simulink model "torqueBalancingStandup"  (Simulink 8.8)
settings: Solver=FixedStepDiscrete  StartTime=0.0  StopTime="Config.SIMULATION_TIME "  FixedStep=Config.Ts  RelTol=1e-3  EnableMultiTasking=on
InitFcn:
  | cd(fileparts(which(bdroot)));
  | initTorqueBalancingStandup;
StopFcn:
  | cd(fileparts(which(bdroot)));
  | stopTorqueBalancingStandup;
undefined symbols (not defined in the file or in its folder): bVectorConstraintsFeet, bVectorConstraintsLegs, Config, ConstraintsMatrixFeet, ConstraintsMatrixLegs, Gain, HUMAN_DOF_FOR_SIMULINK, Reg, ROBOT_DOF, ROBOT_DOF_FOR_SIMULINK, Sat, Sm
libraries: WBToolboxLibrary x128, simulink x4
(part 1 of 3)
settings Model: SuppressorTable=22 serialization::archive 11 0 3 0 0 0 11 0  Creator=daniele  LastModifiedBy=yeshi  NumberOfSteps=100
settings DataIOCC: SignalLoggingSaveFormat=Dataset
settings OptimizationCC: ExpressionDepthLimit=2147483647
settings DebuggingCC: SolverPrmCheckMsg=warning  AllowSymbolicDim=off
settings SFSimCC: SimParseCustomCode=off

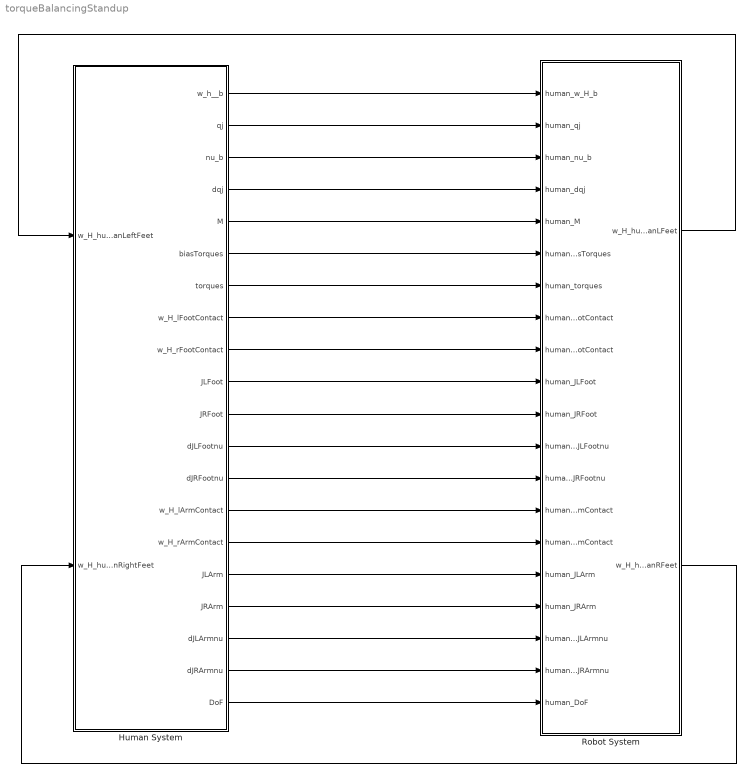
== system torqueBalancingStandup ==
  Human System : Subsystem
  Robot System : Subsystem
  wires:
  Human System/15(w_H_rArmContact) -> Robot System/15(human_w_H_rArmContact)
  Human System/8(w_H_lFootContact) -> Robot System/8(human_w_H_lFootContact)
  Human System/9(w_H_rFootContact) -> Robot System/9(human_w_H_rFootContact)
  Human System/17(JRArm) -> Robot System/17(human_JRArm)
  Human System/19(dJRArmnu) -> Robot System/19(human_dJRArmnu)
  Human System/14(w_H_lArmContact) -> Robot System/14(human_w_H_lArmContact)
  Human System/11(JRFoot) -> Robot System/11(human_JRFoot)
  Human System/12(dJLFootnu) -> Robot System/12(human_dJLFootnu)
  Human System/18(dJLArmnu) -> Robot System/18(human_dJLArmnu)
  Human System/13(dJRFootnu) -> Robot System/13(human_dJRFootnu)
  Human System/1(w_h__b) -> Robot System/1(human_w_H_b)
  Human System/2(qj) -> Robot System/2(human_qj)
  Human System/3(nu_b) -> Robot System/3(human_nu_b)
  Human System/4(dqj) -> Robot System/4(human_dqj)
  Human System/5(M) -> Robot System/5("human_M ")
  Human System/6(biasTorques) -> Robot System/6("human_biasTorques ")
  Human System/10(JLFoot) -> Robot System/10(human_JLFoot)
  Human System/16(JLArm) -> Robot System/16(human_JLArm)
  Human System/7(torques) -> Robot System/7(human_torques)
  Human System/20(DoF) -> Robot System/20(human_DoF)
  Robot System/1(w_H_humanLFeet) -> Human System/1(w_H_humanLeftFeet)
  Robot System/2(w_H_humanRFeet) -> Human System/2(w_H_humanRightFeet)

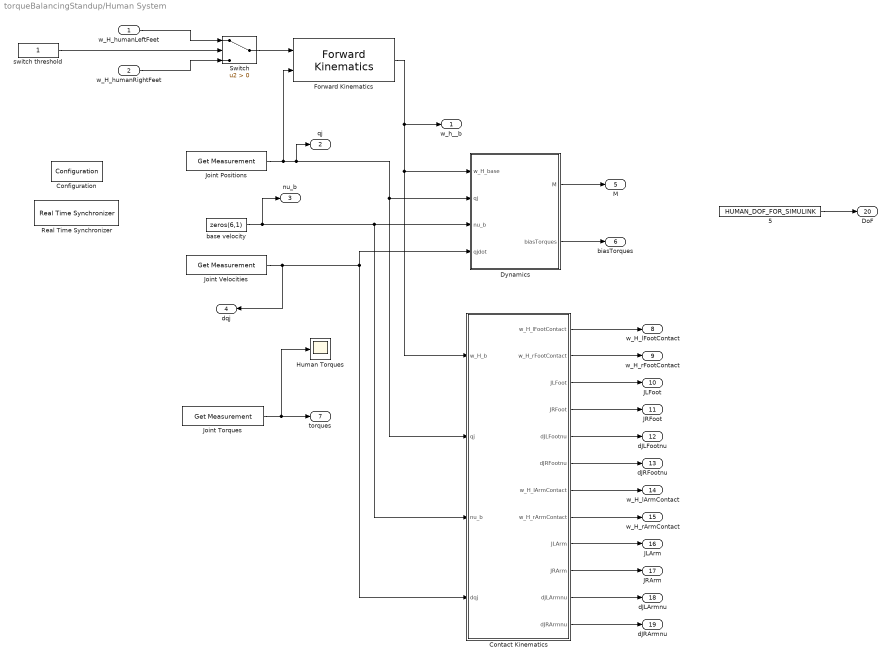
== system torqueBalancingStandup/Human System ==
  w_H_humanLeftFeet : Inport
  w_H_humanRightFeet : Inport  Port=2
  "    5" : Constant  Value=HUMAN_DOF_FOR_SIMULINK
  Configuration : WBToolboxLibrary/Utilities/Configuration  ConfigSource=Workspace  ConfigObject='HUMAN_WBTConfigRobot'
  Contact Kinematics : Subsystem
  Dynamics : Subsystem
  Forward Kinematics : WBToolboxLibrary/wholeBodyModel/Kinematics/Forward Kinematics  frameName=HUMAN_Frames.BASE
  Human Torques : Scope
  Joint Positions : WBToolboxLibrary/wholeBodyStates/Get Measurement  measuredType=Joints Position
  Joint Torques : WBToolboxLibrary/wholeBodyStates/Get Measurement  measuredType=Joints Torque
  Joint Velocities : WBToolboxLibrary/wholeBodyStates/Get Measurement  measuredType=Joints Velocity
  Real Time Synchronizer : WBToolboxLibrary/Utilities/Real Time Synchronizer  period=0.01  mask(Real Time Synchronizer){}
  Switch : Switch  Criteria=u2 > Threshold
  base velocity : Constant  Value=zeros(6,1)
  switch threshold : Constant
  w_h__b : Outport
  qj : Outport  Port=2
  nu_b : Outport  Port=3
  dqj : Outport  Port=4
  M : Outport  Port=5
  biasTorques : Outport  Port=6
  torques : Outport  Port=7
  w_H_lFootContact : Outport  Port=8
  w_H_rFootContact : Outport  Port=9
  JLFoot : Outport  Port=10
  JRFoot : Outport  Port=11
  dJLFootnu : Outport  Port=12
  dJRFootnu : Outport  Port=13
  w_H_lArmContact : Outport  Port=14
  w_H_rArmContact : Outport  Port=15
  JLArm : Outport  Port=16
  JRArm : Outport  Port=17
  dJLArmnu : Outport  Port=18
  dJRArmnu : Outport  Port=19
  DoF : Outport  Port=20
  wires:
  Joint Positions/1 -> Dynamics/2(qj), Contact Kinematics/2(qj), qj/1, Forward Kinematics/2
  base velocity/1 -> nu_b/1, Dynamics/3(nu_b), Contact Kinematics/3(nu_b)
  Joint Velocities/1 -> dqj/1, Dynamics/4(qjdot), Contact Kinematics/4(dqj)
  Forward Kinematics/1 -> w_h__b/1, Contact Kinematics/1(w_H_b), Dynamics/1(w_H_base)
  Dynamics/1(M) -> M/1
  Dynamics/2(biasTorques) -> biasTorques/1
  Contact Kinematics/1(w_H_lFootContact) -> w_H_lFootContact/1
  Contact Kinematics/2(w_H_rFootContact) -> w_H_rFootContact/1
  Contact Kinematics/3(JLFoot) -> JLFoot/1
  Contact Kinematics/4(JRFoot) -> JRFoot/1
  Contact Kinematics/5(dJLFootnu) -> dJLFootnu/1
  Contact Kinematics/6(dJRFootnu) -> dJRFootnu/1
  Contact Kinematics/7(w_H_lArmContact) -> w_H_lArmContact/1
  Contact Kinematics/8(w_H_rArmContact) -> w_H_rArmContact/1
  Contact Kinematics/9(JLArm) -> JLArm/1
  Contact Kinematics/10(JRArm) -> JRArm/1
  Contact Kinematics/11(dJLArmnu) -> dJLArmnu/1
  Contact Kinematics/12(dJRArmnu) -> dJRArmnu/1
  Joint Torques/1 -> Human Torques/1, torques/1
  "    5"/1 -> DoF/1
  w_H_humanRightFeet/1 -> Switch/3
  Switch/1 -> Forward Kinematics/1
  w_H_humanLeftFeet/1 -> Switch/1
  switch threshold/1 -> Switch/2

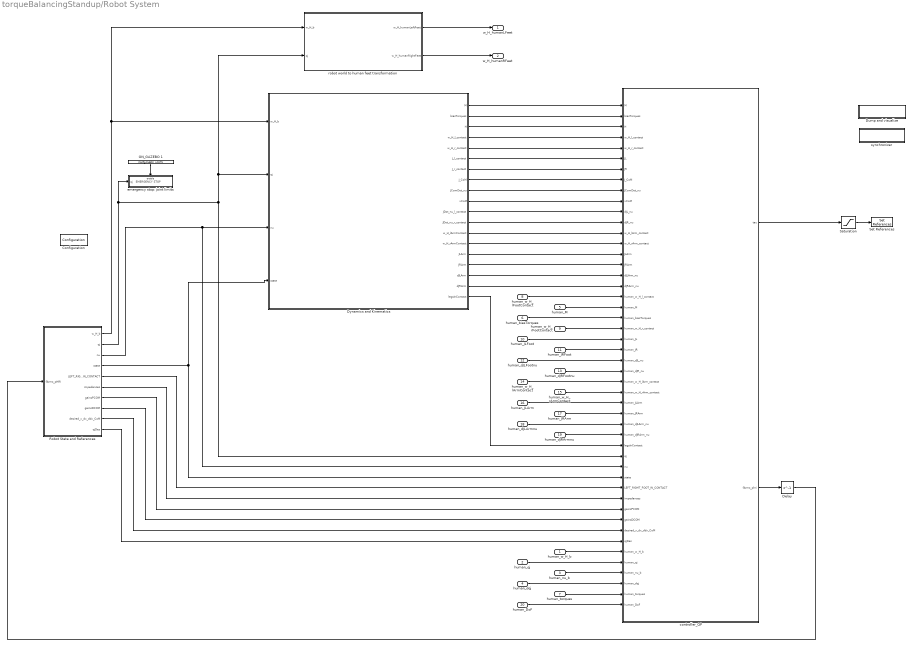
== system torqueBalancingStandup/Robot System ==
  human_w_H_b : Inport
  human_qj : Inport  Port=2
  human_nu_b : Inport  Port=3
  human_dqj : Inport  Port=4
  "human_M " : Inport  Port=5
  "human_biasTorques " : Inport  Port=6
  human_torques : Inport  Port=7
  human_w_H_lFootContact : Inport  Port=8
  human_w_H_rFootContact : Inport  Port=9
  human_JLFoot : Inport  Port=10
  human_JRFoot : Inport  Port=11
  human_dJLFootnu : Inport  Port=12
  human_dJRFootnu : Inport  Port=13
  human_w_H_lArmContact : Inport  Port=14
  human_w_H_rArmContact : Inport  Port=15
  human_JLArm : Inport  Port=16
  human_JRArm : Inport  Port=17
  human_dJLArmnu : Inport  Port=18
  human_dJRArmnu : Inport  Port=19
  human_DoF : Inport  Port=20
  Configuration : WBToolboxLibrary/Utilities/Configuration  ConfigSource=Workspace  ConfigObject='WBTConfigRobot'
  Delay : Delay  DelayLength=1
  Dump and visualize : Subsystem
      mask Display: disp('VISUALIZER')
  Dynamics and Kinematics : Subsystem
  ON_GAZEBO 1 : Constant  Value=Config.CHECK_LIMITS
  Robot State and References : Subsystem  Priority=-10
  Saturation : Saturate  UpperLimit=Sat.torque  LowerLimit=-Sat.torque
  Set References : WBToolboxLibrary/wholeBodyActuators/Set References  controlType=Torque  refSpeed=50
  controller_QP : Subsystem
  emergency stop: joint limits : Subsystem
  robot world to human feet transformation : Subsystem
  synchronizer : Subsystem
      mask Display: disp('SYNCHRONIZER')
  w_H_humanLFeet : Outport
  w_H_humanRFeet : Outport  Port=2
  wires:
  ON_GAZEBO 1/1 -> emergency stop: joint limits/Enable
  Saturation/1 -> Set References/1
  Robot State and References/2(qj) -> controller_QP/34(qj), Dynamics and Kinematics/2(qj), robot world to human feet transformation/2(qj), emergency stop: joint limits/1(qj   EMERGENCY STOP)
  Robot State and References/3(nu) -> Dynamics and Kinematics/3(nu), controller_QP/35(nu)
  Robot State and References/4(state) -> controller_QP/36(state), Dynamics and Kinematics/4("state ")
  Robot State and References/1(w_H_b) -> robot world to human feet transformation/1(w_H_b), Dynamics and Kinematics/1(w_H_b)
  Dynamics and Kinematics/1(M) -> controller_QP/1(M)
  "human_M "/1 -> controller_QP/20(human_M)
  "human_biasTorques "/1 -> controller_QP/21(human_biasTorques)
  Dynamics and Kinematics/2(biasTorques) -> controller_QP/2(biasTorques)
  Dynamics and Kinematics/3(H) -> controller_QP/3("H ")
  Dynamics and Kinematics/4(w_H_l_contact) -> controller_QP/4(w_H_l_contact)
  Dynamics and Kinematics/5(w_H_r_contact) -> controller_QP/5(w_H_r_contact)
  Dynamics and Kinematics/6(J_l_contact) -> controller_QP/6(JL)
  Dynamics and Kinematics/7(J_r_contact) -> controller_QP/7(JR)
  Dynamics and Kinematics/8(J_CoM) -> controller_QP/8(J_CoM)
  Dynamics and Kinematics/10(xCoM) -> controller_QP/10(xCoM)
  Dynamics and Kinematics/11(JDot_nu_l_contact) -> controller_QP/11(dJL_nu)
  Dynamics and Kinematics/12(JDot_nu_r_contact) -> controller_QP/12(dJR_nu)
  Dynamics and Kinematics/13(w_H_lArmContact) -> controller_QP/13(w_H_lArm_contact)
  Dynamics and Kinematics/14(w_H_rArmContact) -> controller_QP/14(w_H_rArm_contact)
  Dynamics and Kinematics/15(JLArm) -> controller_QP/15(JLArm)
  Dynamics and Kinematics/16(JRArm) -> controller_QP/16(JRArm)
  Dynamics and Kinematics/17(dJLArm) -> controller_QP/17(dJLArm_nu)
  Dynamics and Kinematics/18(dJRArm) -> controller_QP/18(dJRArm_nu)
  Dynamics and Kinematics/19(legsInContact) -> controller_QP/33(legsInContact)
  human_w_H_lFootContact/1 -> controller_QP/19(human_w_H_l_contact)
  human_w_H_rFootContact/1 -> controller_QP/22(human_w_H_r_contact)
  human_JLFoot/1 -> controller_QP/23(human_JL)
  human_JRFoot/1 -> controller_QP/24(human_JR)
  human_dJLFootnu/1 -> controller_QP/25(human_dJL_nu)
  human_dJRFootnu/1 -> controller_QP/26(human_dJR_nu)
  human_w_H_lArmContact/1 -> controller_QP/27(human_w_H_lArm_contact)
  human_w_H_rArmContact/1 -> controller_QP/28(human_w_H_rArm_contact)
  human_JLArm/1 -> controller_QP/29(human_JLArm)
  human_JRArm/1 -> controller_QP/30(human_JRArm)
  human_dJLArmnu/1 -> controller_QP/31(human_dJLArm_nu)
  human_dJRArmnu/1 -> controller_QP/32(human_dJRArm_nu)
  controller_QP/1("tau ") -> Saturation/1
  Robot State and References/5(LEFT_RIGHT_FOOT_IN_CONTACT) -> controller_QP/37(LEFT_RIGHT_FOOT_IN_CONTACT)
  Robot State and References/6(impedances) -> controller_QP/38(impedances)
  Robot State and References/7(gainsPCOM) -> controller_QP/39(gainsPCOM)
  Robot State and References/8(gainsDCOM) -> controller_QP/40(gainsDCOM)
  Robot State and References/9(desired_x_dx_ddx_CoM) -> controller_QP/41(desired_x_dx_ddx_CoM)
  Robot State and References/10(qjDes) -> controller_QP/42(qjDes)
  human_w_H_b/1 -> controller_QP/43(human_w_H_b)
  human_qj/1 -> controller_QP/44(human_qj)
  human_nu_b/1 -> controller_QP/45(human_nu_b)
  human_dqj/1 -> controller_QP/46(human_dqj)
  human_torques/1 -> controller_QP/47(human_torques)
  human_DoF/1 -> controller_QP/48(human_DoF)
  robot world to human feet transformation/1(w_H_humanLeftFeet) -> w_H_humanLFeet/1
  robot world to human feet transformation/2(w_H_humanRightFeet) -> w_H_humanRFeet/1
  Dynamics and Kinematics/9(JComDot_nu) -> controller_QP/9(JComDot_nu)
  controller_QP/2(fArms_phri) -> Delay/1
  Delay/1 -> Robot State and References/1(fArms_pHRI)

== system torqueBalancingStandup/Human System/Contact Kinematics ==
  w_H_b : Inport
  qj : Inport  Port=2
  nu_b : Inport  Port=3
  dqj : Inport  Port=4
  Arm Contacts Kinematics : Subsystem
  Leg Contacts Kinematics : Subsystem
  w_H_lFootContact : Outport
  w_H_rFootContact : Outport  Port=2
  JLFoot : Outport  Port=3
  JRFoot : Outport  Port=4
  dJLFootnu : Outport  Port=5
  dJRFootnu : Outport  Port=6
  w_H_lArmContact : Outport  Port=7
  w_H_rArmContact : Outport  Port=8
  JLArm : Outport  Port=9
  JRArm : Outport  Port=10
  dJLArmnu : Outport  Port=11
  dJRArmnu : Outport  Port=12
  wires:
  Arm Contacts Kinematics/3(JLArm) -> JLArm/1
  Arm Contacts Kinematics/5(dJLArmnu) -> dJLArmnu/1
  Leg Contacts Kinematics/3(JLFoot) -> JLFoot/1
  Arm Contacts Kinematics/6(dJRArmnu) -> dJRArmnu/1
  w_H_b/1 -> Arm Contacts Kinematics/1(w_H_b1), Leg Contacts Kinematics/1(w_H_b1)
  nu_b/1 -> Arm Contacts Kinematics/3(nu_b), Leg Contacts Kinematics/3(nu_b)
  Leg Contacts Kinematics/1(w_H_lFootContact) -> w_H_lFootContact/1
  Leg Contacts Kinematics/6(dJRFootnu) -> dJRFootnu/1
  Leg Contacts Kinematics/4(JRFoot) -> JRFoot/1
  Leg Contacts Kinematics/5(dJLFootnu) -> dJLFootnu/1
  Arm Contacts Kinematics/1(w_H_lArmContact) -> w_H_lArmContact/1
  dqj/1 -> Arm Contacts Kinematics/4(dqj), Leg Contacts Kinematics/4(dqj)
  Leg Contacts Kinematics/2(w_H_rFootContact) -> w_H_rFootContact/1
  Arm Contacts Kinematics/2(w_H_rArmContact) -> w_H_rArmContact/1
  Arm Contacts Kinematics/4(JRArm) -> JRArm/1
  qj/1 -> Arm Contacts Kinematics/2(qj1), Leg Contacts Kinematics/2(qj1)

== system torqueBalancingStandup/Human System/Dynamics ==
  w_H_base : Inport
  qj : Inport  Port=2
  nu_b : Inport  Port=3
  qjdot : Inport  Port=4
  Get Bias Forces : WBToolboxLibrary/wholeBodyModel/Dynamics/Get Bias Forces
  Mass Matrix : WBToolboxLibrary/wholeBodyModel/Dynamics/Mass Matrix
  M : Outport
  biasTorques : Outport  Port=2
  wires:
  Get Bias Forces/1 -> biasTorques/1
  w_H_base/1 -> Get Bias Forces/1, Mass Matrix/1
  qj/1 -> Get Bias Forces/2, Mass Matrix/2
  nu_b/1 -> Get Bias Forces/3
  Mass Matrix/1 -> M/1
  qjdot/1 -> Get Bias Forces/4

== system torqueBalancingStandup/Robot System/Dump and visualize ==
  Human assistance : Subsystem
  Logical Operator1 : Logic  Operator=OR  AllPortsSameDT=off  OutDataTypeStr=boolean
  ON_GAZEBO 3 : Constant  Value=Config.SCOPES_ALL
  ON_GAZEBO 4 : Constant  Value=Config.SCOPES_MAIN
  Robot data : Subsystem
  wires:
  ON_GAZEBO 3/1 -> Logical Operator1/1
  ON_GAZEBO 4/1 -> Logical Operator1/2
  Logical Operator1/1 -> Robot data/Enable
  [CoM_error] -> Robot data/5(CoM_Error)
  [f_QP] -> Robot data/6(fDesQP)
  [f_noQP] -> Robot data/8(fDesNoQP)
  [qj_des] -> Robot data/4(qj_des)
  [w_H_b] -> Robot data/2(w_H_b)
  [tau_des] -> Robot data/1(tau_des)
  [CoM_des] -> Robot data/7(CoM_des)
  [state] -> Human assistance/1(state), Robot data/3(state)

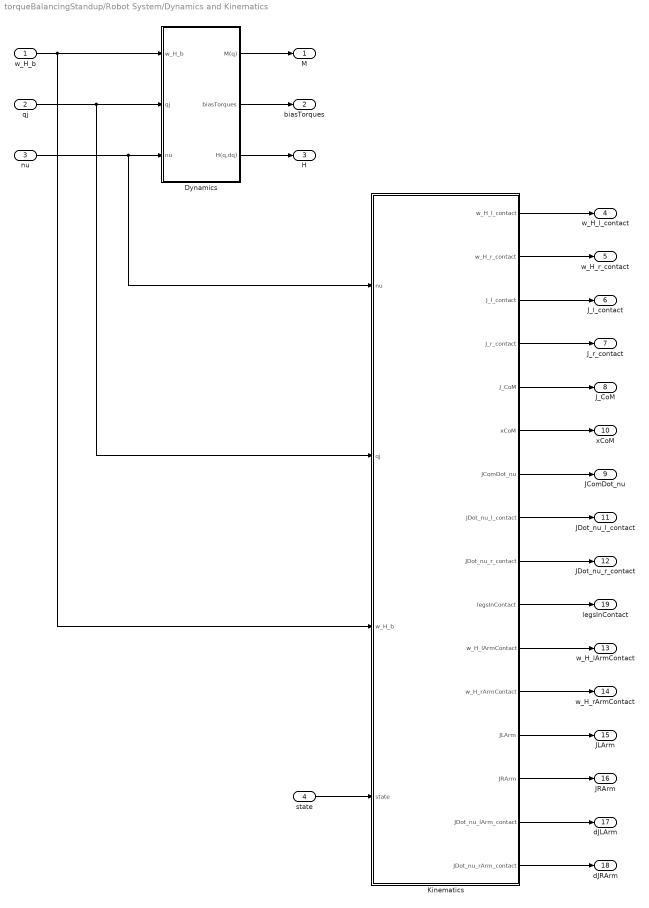
== system torqueBalancingStandup/Robot System/Dynamics and Kinematics ==
  w_H_b : Inport
  qj : Inport  Port=2
  nu : Inport  Port=3
  "state " : Inport  Port=4
  Dynamics : Subsystem
  Kinematics : Subsystem
  M : Outport
  biasTorques : Outport  Port=2
  H : Outport  Port=3
  w_H_l_contact : Outport  Port=4
  w_H_r_contact : Outport  Port=5
  J_l_contact : Outport  Port=6
  J_r_contact : Outport  Port=7
  J_CoM : Outport  Port=8
  JComDot_nu : Outport  Port=9
  xCoM : Outport  Port=10
  JDot_nu_l_contact : Outport  Port=11
  JDot_nu_r_contact : Outport  Port=12
  w_H_lArmContact : Outport  Port=13
  w_H_rArmContact : Outport  Port=14
  JLArm : Outport  Port=15
  JRArm : Outport  Port=16
  dJLArm : Outport  Port=17
  dJRArm : Outport  Port=18
  legsInContact : Outport  Port=19
  wires:
  w_H_b/1 -> Kinematics/3(w_H_b), Dynamics/1(w_H_b)
  qj/1 -> Dynamics/2(qj), Kinematics/2(qj)
  nu/1 -> Dynamics/3(nu), Kinematics/1(nu)
  Dynamics/1(M(q)) -> M/1
  Dynamics/2(biasTorques) -> biasTorques/1
  Dynamics/3(H(q,dq)) -> H/1
  Kinematics/5(J_CoM) -> J_CoM/1
  Kinematics/6(xCoM) -> xCoM/1
  Kinematics/1(w_H_l_contact) -> w_H_l_contact/1
  Kinematics/2(w_H_r_contact) -> w_H_r_contact/1
  Kinematics/8(JDot_nu_l_contact) -> JDot_nu_l_contact/1
  Kinematics/9(JDot_nu_r_contact) -> JDot_nu_r_contact/1
  Kinematics/3(J_l_contact) -> J_l_contact/1
  Kinematics/4(J_r_contact) -> J_r_contact/1
  Kinematics/10(legsInContact) -> legsInContact/1
  "state "/1 -> Kinematics/4("state ")
  Kinematics/11(w_H_lArmContact) -> w_H_lArmContact/1
  Kinematics/12(w_H_rArmContact) -> w_H_rArmContact/1
  Kinematics/13(JLArm) -> JLArm/1
  Kinematics/14(JRArm) -> JRArm/1
  Kinematics/15(JDot_nu_lArm_contact) -> dJLArm/1
  Kinematics/16(JDot_nu_rArm_contact) -> dJRArm/1
  Kinematics/7(JComDot_nu) -> JComDot_nu/1

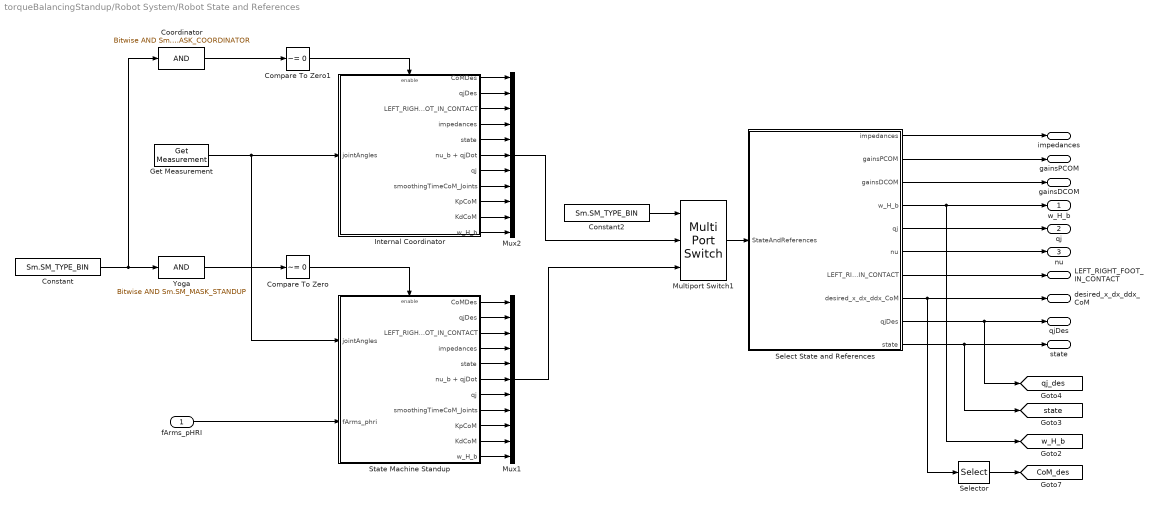
== system torqueBalancingStandup/Robot System/Robot State and References ==
  fArms_pHRI : Inport
  Compare To Zero : simulink/Logic and Bit Operations/Compare To Zero  relop=~=  OutDataTypeStr=boolean
  Compare To Zero1 : simulink/Logic and Bit Operations/Compare To Zero  relop=~=  OutDataTypeStr=boolean
  Constant : Constant  Priority=-10  Value=Sm.SM_TYPE_BIN  OutDataTypeStr=uint8
  Constant2 : Constant  Priority=-10  Value=Sm.SM_TYPE_BIN  OutDataTypeStr=uint8
  Coordinator : simulink/Logic and Bit Operations/Bitwise Operator  logicop=AND  UseBitMask=on  BitMask=Sm.SM_MASK_COORDINATOR  BitMaskRealWorld=Stored Integer
  Get Measurement : WBToolboxLibrary/wholeBodyStates/Get Measurement  measuredType=Joints Position
  Internal Coordinator : Subsystem
  Multiport Switch1 : MultiPortSwitch  DataPortOrder=Specify indices  DataPortIndices={1, 2}
  Mux1 : Mux  Inputs=11
  Mux2 : Mux  Inputs=11
  Select State and References : Subsystem
  Selector : Selector  NumberOfDimensions=2  InputPortWidth=3  IndexOptions=Index vector (dialog),Index vector (dialog)  Indices=[1 2 3],[1]  OutputSizes=1,1
  State Machine Standup : Subsystem  Priority=-100
  Yoga : simulink/Logic and Bit Operations/Bitwise Operator  logicop=AND  UseBitMask=on  BitMask=Sm.SM_MASK_STANDUP  BitMaskRealWorld=Stored Integer
  w_H_b : Outport
  qj : Outport  Port=2
  nu : Outport  Port=3
  state : Outport  Port=4
  LEFT_RIGHT_FOOT_IN_CONTACT : Outport  Port=5
  impedances : Outport  Port=6
  gainsPCOM : Outport  Port=7
  gainsDCOM : Outport  Port=8
  desired_x_dx_ddx_CoM : Outport  Port=9
  qjDes : Outport  Port=10
  tag scope: CoM_des=global, qj_des=global, state=global, w_H_b=global
  wires:
  Constant/1 -> Yoga/1, Coordinator/1
  State Machine Standup/3(LEFT_RIGHT_FOOT_IN_CONTACT) -> Mux1/3
  State Machine Standup/2(qjDes) -> Mux1/2
  State Machine Standup/1(CoMDes) -> Mux1/1
  Internal Coordinator/1(CoMDes) -> Mux2/1
  Internal Coordinator/2(qjDes) -> Mux2/2
  Internal Coordinator/3(LEFT_RIGHT_FOOT_IN_CONTACT) -> Mux2/3
  State Machine Standup/4(impedances) -> Mux1/4
  Internal Coordinator/4(impedances) -> Mux2/4
  State Machine Standup/5(state) -> Mux1/5
  Internal Coordinator/5(state) -> Mux2/5
  Internal Coordinator/6(nu_b + qjDot) -> Mux2/6
  Internal Coordinator/7(qj) -> Mux2/7
  State Machine Standup/6(nu_b + qjDot) -> Mux1/6
  State Machine Standup/7(qj) -> Mux1/7
  Coordinator/1 -> Compare To Zero1/1
  Yoga/1 -> Compare To Zero/1
  Compare To Zero/1 -> State Machine Standup/Enable
  Compare To Zero1/1 -> Internal Coordinator/Enable
  Internal Coordinator/8(smoothingTimeCoM_Joints) -> Mux2/8
  State Machine Standup/8(smoothingTimeCoM_Joints) -> Mux1/8
  State Machine Standup/9(KpCoM) -> Mux1/9
  State Machine Standup/10(KdCoM) -> Mux1/10
  Internal Coordinator/9(KpCoM) -> Mux2/9
  Internal Coordinator/10(KdCoM) -> Mux2/10
  Constant2/1 -> Multiport Switch1/1
  Get Measurement/1 -> Internal Coordinator/1(jointAngles), State Machine Standup/1(jointAngles)
  State Machine Standup/11(w_H_b) -> Mux1/11
  Internal Coordinator/11(w_H_b) -> Mux2/11
  Mux2/1 -> Multiport Switch1/2
  Multiport Switch1/1 -> Select State and References/1(StateAndReferences)
  Select State and References/1(impedances) -> impedances/1
  Select State and References/2(gainsPCOM) -> gainsPCOM/1
  Select State and References/3(gainsDCOM) -> gainsDCOM/1
  Select State and References/4(w_H_b) -> w_H_b/1, [w_H_b]
  Select State and References/5(qj) -> qj/1
  Select State and References/6(nu) -> nu/1
  Select State and References/7(LEFT_RIGHT_FOOT_IN_CONTACT) -> LEFT_RIGHT_FOOT_IN_CONTACT/1
  Select State and References/8(desired_x_dx_ddx_CoM) -> desired_x_dx_ddx_CoM/1, Selector/1
  Select State and References/9(qjDes) -> qjDes/1, [qj_des]
  Select State and References/10(state) -> state/1, [state]
  Selector/1 -> [CoM_des]
  Mux1/1 -> Multiport Switch1/3
  fArms_pHRI/1 -> State Machine Standup/2(fArms_phri)

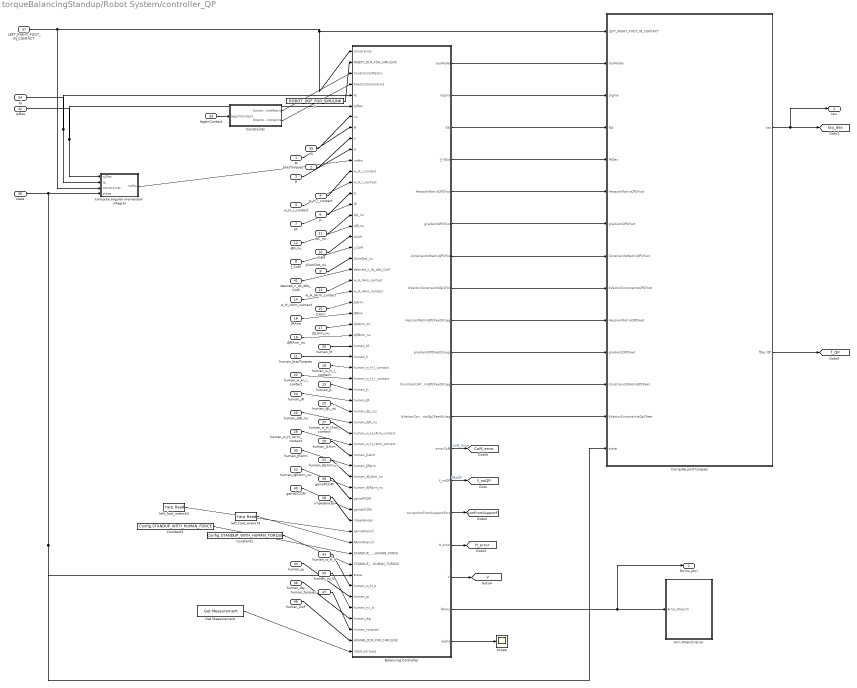
== system torqueBalancingStandup/Robot System/controller_QP ==
  M : Inport
  biasTorques : Inport  Port=2
  "H " : Inport  Port=3
  w_H_l_contact : Inport  Port=4
  w_H_r_contact : Inport  Port=5
  JL : Inport  Port=6
  JR : Inport  Port=7
  J_CoM : Inport  Port=8
  JComDot_nu : Inport  Port=9
  xCoM : Inport  Port=10
  dJL_nu : Inport  Port=11
  dJR_nu : Inport  Port=12
  w_H_lArm_contact : Inport  Port=13
  w_H_rArm_contact : Inport  Port=14
  JLArm : Inport  Port=15
  JRArm : Inport  Port=16
  dJLArm_nu : Inport  Port=17
  dJRArm_nu : Inport  Port=18
  human_w_H_l_contact : Inport  Port=19
  human_M : Inport  Port=20
  human_biasTorques : Inport  Port=21
  human_w_H_r_contact : Inport  Port=22
  human_JL : Inport  Port=23
  human_JR : Inport  Port=24
  human_dJL_nu : Inport  Port=25
  human_dJR_nu : Inport  Port=26
  human_w_H_lArm_contact : Inport  Port=27
  human_w_H_rArm_contact : Inport  Port=28
  human_JLArm : Inport  Port=29
  human_JRArm : Inport  Port=30
  human_dJLArm_nu : Inport  Port=31
  human_dJRArm_nu : Inport  Port=32
  legsInContact : Inport  Port=33
  qj : Inport  Port=34
  nu : Inport  Port=35
  state : Inport  Port=36
  LEFT_RIGHT_FOOT_IN_CONTACT : Inport  Port=37
  impedances : Inport  Port=38
  gainsPCOM : Inport  Port=39
  gainsDCOM : Inport  Port=40
  desired_x_dx_ddx_CoM : Inport  Port=41
  qjDes : Inport  Port=42
  human_w_H_b : Inport  Port=43
  human_qj : Inport  Port=44
  human_nu_b : Inport  Port=45
  human_dqj : Inport  Port=46
  human_torques : Inport  Port=47
  human_DoF : Inport  Port=48
  "    5" : Constant  Value=ROBOT_DOF_FOR_SIMULINK
  Arm Wrench Error : Subsystem
  "Balancing Controller " : MATLAB Function  TreatAsAtomicUnit=on
  Compute angular momentum integral : Subsystem
  Compute joint torques : Subsystem
  Constant1 : Constant  Value=Config.STANDUP_WITH_HUMAN_TORQUE
  Constant2 : Constant  Value=Config.STANDUP_WITH_HUMAN_FORCE
  Constraints : Subsystem
  Get Measurement : WBToolboxLibrary/wholeBodyStates/Get Measurement  measuredType=Joints Torque
  Scope : Scope
  left_foot_wrench1 : WBToolboxLibrary/Utilities/Yarp Read  portName=Ports.RIGHT_ARM  signalSize=6  timeout=0.5  blocking=off  timestamp=off  autoconnect=on  errorOnConnection=on
  left_foot_wrench2 : WBToolboxLibrary/Utilities/Yarp Read  portName=Ports.LEFT_ARM  signalSize=6  timeout=0.5  blocking=off  timestamp=off  autoconnect=on  errorOnConnection=on
  "tau " : Outport
  fArms_phri : Outport  Port=2
  tag scope: CoM_error=global, H_error=global, V=global, corrFromSupportF=global, f_QP=global, f_noQP=global, tau_des=global
  wires:
  qj/1 -> "Balancing Controller "/5(qj), Compute angular momentum integral/2(qj)
  qjDes/1 -> Compute angular momentum integral/1(qjDes), "Balancing Controller "/6(qjDes)
  legsInContact/1 -> Constraints/1(legsInContact)
  M/1 -> "Balancing Controller "/8(M)
  human_M/1 -> "Balancing Controller "/28(human_M)
  biasTorques/1 -> "Balancing Controller "/9(h)
  human_biasTorques/1 -> "Balancing Controller "/29(human_h)
  "H "/1 -> "Balancing Controller "/10(H)
  Compute angular momentum integral/1(intHw) -> "Balancing Controller "/11(intHw)
  w_H_l_contact/1 -> "Balancing Controller "/12(w_H_l_contact)
  w_H_r_contact/1 -> "Balancing Controller "/13(w_H_r_contact)
  JL/1 -> "Balancing Controller "/14(JL)
  JR/1 -> "Balancing Controller "/15(JR)
  dJL_nu/1 -> "Balancing Controller "/16(dJL_nu)
  dJR_nu/1 -> "Balancing Controller "/17(dJR_nu)
  xCoM/1 -> "Balancing Controller "/18(xCoM)
  J_CoM/1 -> "Balancing Controller "/19(J_CoM)
  desired_x_dx_ddx_CoM/1 -> "Balancing Controller "/21(desired_x_dx_ddx_CoM)
  w_H_lArm_contact/1 -> "Balancing Controller "/22(w_H_lArm_contact)
  w_H_rArm_contact/1 -> "Balancing Controller "/23(w_H_rArm_contact)
  JLArm/1 -> "Balancing Controller "/24(JLArm)
  JRArm/1 -> "Balancing Controller "/25(JRArm)
  dJLArm_nu/1 -> "Balancing Controller "/26(dJLArm_nu)
  dJRArm_nu/1 -> "Balancing Controller "/27(dJRArm_nu)
  human_w_H_l_contact/1 -> "Balancing Controller "/30(human_w_H_l_contact)
  human_w_H_r_contact/1 -> "Balancing Controller "/31(human_w_H_r_contact)
  human_JL/1 -> "Balancing Controller "/32(human_JL)
  human_JR/1 -> "Balancing Controller "/33(human_JR)
  human_dJL_nu/1 -> "Balancing Controller "/34(human_dJL_nu)
  human_dJR_nu/1 -> "Balancing Controller "/35(human_dJR_nu)
  human_w_H_lArm_contact/1 -> "Balancing Controller "/36(human_w_H_lArm_contact)
  human_w_H_rArm_contact/1 -> "Balancing Controller "/37(human_w_H_rArm_contact)
  human_JLArm/1 -> "Balancing Controller "/38(human_JLArm)
  human_JRArm/1 -> "Balancing Controller "/39(human_JRArm)
  human_dJLArm_nu/1 -> "Balancing Controller "/40(human_dJLArm_nu)
  human_dJRArm_nu/1 -> "Balancing Controller "/41(human_dJRArm_nu)
  gainsPCOM/1 -> "Balancing Controller "/42(gainsPCOM)
  gainsDCOM/1 -> "Balancing Controller "/43(gainsDCOM)
  impedances/1 -> "Balancing Controller "/44(impedances)
  left_foot_wrench2/1 -> "Balancing Controller "/45(LArmWrench)
  left_foot_wrench1/1 -> "Balancing Controller "/46(RArmWrench)
  Constant2/1 -> "Balancing Controller "/47(STANDUP_WITH_HUMAN_FORCE)
  nu/1 -> "Balancing Controller "/7(nu)
  Constraints/2(bVectorConstraints) -> "Balancing Controller "/4(bVectorConstraints)
  Constraints/1(ConstraintsMatrix) -> "Balancing Controller "/3(ConstraintsMatrix)
  "    5"/1 -> "Balancing Controller "/2(ROBOT_DOF_FOR_SIMULINK)
  "Balancing Controller "/13(errorCoM) -> [CoM_error]  "CoM_Error"
  "Balancing Controller "/14(f_noQP) -> [f_noQP]  "fNoQP"
  "Balancing Controller "/15(correctionFromSupportForce) -> [corrFromSupportF]
  "Balancing Controller "/16(H_error) -> [H_error]
  "Balancing Controller "/17(V) -> [V]
  human_w_H_b/1 -> "Balancing Controller "/50(human_w_H_b)
  human_qj/1 -> "Balancing Controller "/51(human_qj)
  human_nu_b/1 -> "Balancing Controller "/52(human_nu_b)
  human_dqj/1 -> "Balancing Controller "/53(human_dqj)
  human_torques/1 -> "Balancing Controller "/54(human_torques)
  "Balancing Controller "/1(tauModel) -> Compute joint torques/2(tauModel)
  "Balancing Controller "/2(Sigma) -> Compute joint torques/3(Sigma)
  "Balancing Controller "/3(NA) -> Compute joint torques/4(NA)
  "Balancing Controller "/4(f_HDot) -> Compute joint torques/5(fHDes)
  "Balancing Controller "/5(HessianMatrixQP1Foot) -> Compute joint torques/6(HessianMatrixQP1Foot)
  "Balancing Controller "/6(gradientQP1Foot) -> Compute joint torques/7(gradientQP1Foot)
  "Balancing Controller "/7(ConstraintsMatrixQP1Foot) -> Compute joint torques/8(ConstraintsMatrixQP1Foot)
  "Balancing Controller "/8(bVectorConstraintsQp1Foot) -> Compute joint torques/9(bVectorConstraintsQP1Foot)
  "Balancing Controller "/9(HessianMatrixQP2FeetOrLegs) -> Compute joint torques/10(HessianMatrixQP2Feet)
  "Balancing Controller "/10(gradientQP2FeetOrLegs) -> Compute joint torques/11(gradientQP2Feet)
  "Balancing Controller "/11(ConstraintsMatrixQP2FeetOrLegs) -> Compute joint torques/12(ConstraintsMatrixQP2Feet)
  "Balancing Controller "/12(bVectorConstraintsQp2FeetOrLegs) -> Compute joint torques/13(bVectorConstraintsQp2Feet)
  Compute joint torques/1("tau ") -> "tau "/1, [tau_des]
  Compute joint torques/2(fDes QP) -> [f_QP]
  LEFT_RIGHT_FOOT_IN_CONTACT/1 -> "Balancing Controller "/1(constraints), Compute joint torques/1(LEFT_RIGHT_FOOT_IN_CONTACT), Compute angular momentum integral/3(constraints)
  state/1 -> Compute joint torques/14(state), "Balancing Controller "/49(state), Compute angular momentum integral/4(state)
  human_DoF/1 -> "Balancing Controller "/55(HUMAN_DOF_FOR_SIMULINK)
  Constant1/1 -> "Balancing Controller "/48(STANDUP_WITH_HUMAN_TORQUE)
  JComDot_nu/1 -> "Balancing Controller "/20(JComDot_nu)
  Get Measurement/1 -> "Balancing Controller "/56(robot_torques)
  "Balancing Controller "/19(alpha) -> Scope/1
  "Balancing Controller "/18(fArms) -> fArms_phri/1, Arm Wrench Error/1(Arms_Wrench)

== system torqueBalancingStandup/Robot System/emergency stop: joint limits ==
  qj   EMERGENCY STOP : Inport
  Enable : EnablePort
  Assertion : Assertion
  Get Limits : WBToolboxLibrary/wholeBodyStates/Get Limits  limitsSource=ControlBoard  limitsType=Position
  MATLAB Function : MATLAB Function  TreatAsAtomicUnit=on
  index1 : Constant  Value=0.01  VectorParams1D=off
  wires:
  Get Limits/1 -> MATLAB Function/1(umin)
  Get Limits/2 -> MATLAB Function/2(umax)
  index1/1 -> MATLAB Function/4(tol)
  qj   EMERGENCY STOP/1 -> MATLAB Function/3(u)
  MATLAB Function/1(inRange) -> Assertion/1

== system torqueBalancingStandup/Robot System/robot world to human feet transformation ==
  w_H_b : Inport
  qj : Inport  Port=2
  Forward Kinematics : WBToolboxLibrary/wholeBodyModel/Kinematics/Forward Kinematics  frameName=Frames.LEFT_LEG
  Forward Kinematics1 : WBToolboxLibrary/wholeBodyModel/Kinematics/Forward Kinematics  frameName=Frames.RIGHT_LEG
  MATLAB Function : MATLAB Function  TreatAsAtomicUnit=on
  w_H_humanLeftFeet : Outport
  w_H_humanRightFeet : Outport  Port=2
  wires:
  MATLAB Function/1(w_H_humanLeftFeet) -> w_H_humanLeftFeet/1
  Forward Kinematics1/1 -> MATLAB Function/2(w_H_robotRightFeet)
  Forward Kinematics/1 -> MATLAB Function/1(w_H_robotLeftFeet)
  qj/1 -> Forward Kinematics1/2, Forward Kinematics/2
  w_H_b/1 -> Forward Kinematics1/1, Forward Kinematics/1
  MATLAB Function/2(w_H_humanRightFeet) -> w_H_humanRightFeet/1

== system torqueBalancingStandup/Robot System/synchronizer ==
  GAZEBO_SYNCHRONIZER : Subsystem
  Logical Operator : Logic  Operator=NOT  AllPortsSameDT=off  OutDataTypeStr=boolean
  "ON_GAZEBO " : Constant  Value=Config.ON_GAZEBO
  REAL_TIME_SYNC : Subsystem
  To Workspace : ToWorkspace  VariableName=yarp_time  SaveFormat=Structure With Time  SampleTime=-1
  Yarp Clock : WBToolboxLibrary/Utilities/Yarp Clock
  wires:
  Logical Operator/1 -> REAL_TIME_SYNC/Enable
  "ON_GAZEBO "/1 -> GAZEBO_SYNCHRONIZER/Enable, Logical Operator/1
  Yarp Clock/1 -> To Workspace/1

== system torqueBalancingStandup/Human System/Contact Kinematics/Arm Contacts Kinematics ==
  w_H_b1 : Inport
  qj1 : Inport  Port=2
  nu_b : Inport  Port=3
  dqj : Inport  Port=4
  " " : WBToolboxLibrary/wholeBodyModel/Jacobians/DotJ Nu  frameName=HUMAN_Frames.RIGHT_HAND
  "DotJ Nu l_sole " : WBToolboxLibrary/wholeBodyModel/Jacobians/DotJ Nu  frameName=HUMAN_Frames.LEFT_HAND
  Jacobian l_sole1 : WBToolboxLibrary/wholeBodyModel/Jacobians/Jacobian  frameName=HUMAN_Frames.LEFT_HAND
  Jacobian r_sole1 : WBToolboxLibrary/wholeBodyModel/Jacobians/Jacobian  frameName=HUMAN_Frames.RIGHT_HAND
  l_sole1 : WBToolboxLibrary/wholeBodyModel/Kinematics/Forward Kinematics  frameName=HUMAN_Frames.LEFT_HAND
  r_sole1 : WBToolboxLibrary/wholeBodyModel/Kinematics/Forward Kinematics  frameName=HUMAN_Frames.RIGHT_HAND
  w_H_lArmContact : Outport
  w_H_rArmContact : Outport  Port=2
  JLArm : Outport  Port=3
  JRArm : Outport  Port=4
  dJLArmnu : Outport  Port=5
  dJRArmnu : Outport  Port=6
  wires:
  w_H_b1/1 -> Jacobian l_sole1/1, " "/1, "DotJ Nu l_sole "/1, Jacobian r_sole1/1, r_sole1/1, l_sole1/1
  r_sole1/1 -> w_H_rArmContact/1
  dqj/1 -> "DotJ Nu l_sole "/4, " "/4
  nu_b/1 -> "DotJ Nu l_sole "/3, " "/3
  " "/1 -> dJRArmnu/1
  l_sole1/1 -> w_H_lArmContact/1
  Jacobian r_sole1/1 -> JRArm/1
  qj1/1 -> Jacobian l_sole1/2, " "/2, "DotJ Nu l_sole "/2, Jacobian r_sole1/2, r_sole1/2, l_sole1/2
  Jacobian l_sole1/1 -> JLArm/1
  "DotJ Nu l_sole "/1 -> dJLArmnu/1

== system torqueBalancingStandup/Human System/Contact Kinematics/Leg Contacts Kinematics ==
  w_H_b1 : Inport
  qj1 : Inport  Port=2
  nu_b : Inport  Port=3
  dqj : Inport  Port=4
  " " : WBToolboxLibrary/wholeBodyModel/Jacobians/DotJ Nu  frameName=HUMAN_Frames.RIGHT_FOOT
  "DotJ Nu l_sole " : WBToolboxLibrary/wholeBodyModel/Jacobians/DotJ Nu  frameName=HUMAN_Frames.LEFT_FOOT
  Jacobian l_sole1 : WBToolboxLibrary/wholeBodyModel/Jacobians/Jacobian  frameName=HUMAN_Frames.LEFT_FOOT
  Jacobian r_sole1 : WBToolboxLibrary/wholeBodyModel/Jacobians/Jacobian  frameName=HUMAN_Frames.RIGHT_FOOT
  l_sole1 : WBToolboxLibrary/wholeBodyModel/Kinematics/Forward Kinematics  frameName=HUMAN_Frames.LEFT_FOOT
  r_sole1 : WBToolboxLibrary/wholeBodyModel/Kinematics/Forward Kinematics  frameName=HUMAN_Frames.RIGHT_FOOT
  w_H_lFootContact : Outport
  w_H_rFootContact : Outport  Port=2
  JLFoot : Outport  Port=3
  JRFoot : Outport  Port=4
  dJLFootnu : Outport  Port=5
  dJRFootnu : Outport  Port=6
  wires:
  w_H_b1/1 -> Jacobian l_sole1/1, " "/1, "DotJ Nu l_sole "/1, Jacobian r_sole1/1, r_sole1/1, l_sole1/1
  r_sole1/1 -> w_H_rFootContact/1
  dqj/1 -> "DotJ Nu l_sole "/4, " "/4
  nu_b/1 -> "DotJ Nu l_sole "/3, " "/3
  " "/1 -> dJRFootnu/1
  l_sole1/1 -> w_H_lFootContact/1
  Jacobian r_sole1/1 -> JRFoot/1
  qj1/1 -> Jacobian l_sole1/2, " "/2, "DotJ Nu l_sole "/2, Jacobian r_sole1/2, r_sole1/2, l_sole1/2
  Jacobian l_sole1/1 -> JLFoot/1
  "DotJ Nu l_sole "/1 -> dJLFootnu/1

== system torqueBalancingStandup/Robot System/Dump and visualize/Human assistance ==
  state : Inport
  Htilde : Scope  NumInputPorts=2
  V_lyap : Scope  NumInputPorts=2
  humanSupport6DForce : Scope  NumInputPorts=2
  wires:
  [H_error] -> Htilde/1
  state/1 -> V_lyap/2, Htilde/2, humanSupport6DForce/2
  [corrFromSupportF] -> humanSupport6DForce/1
  [V] -> V_lyap/1

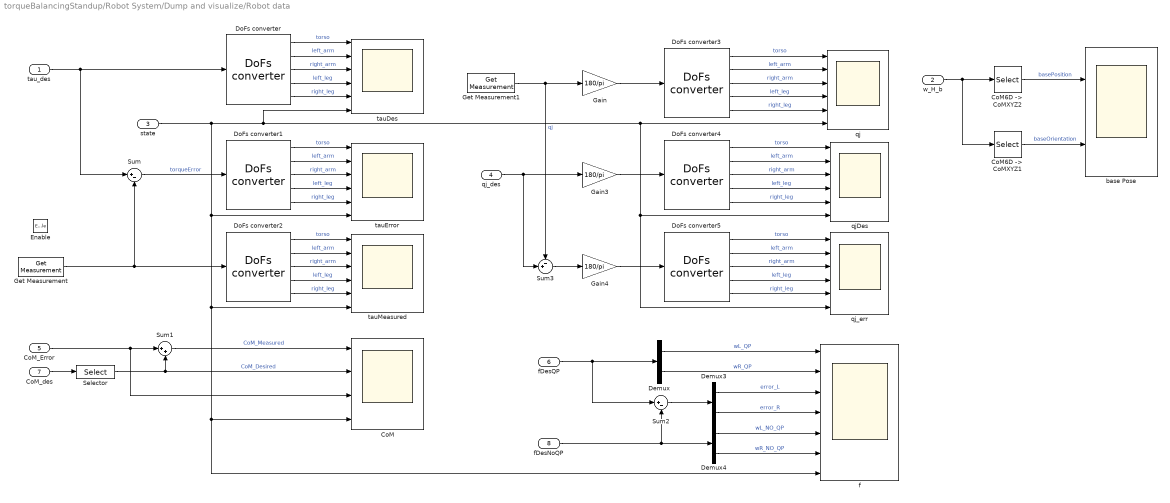
== system torqueBalancingStandup/Robot System/Dump and visualize/Robot data ==
  tau_des : Inport
  w_H_b : Inport  Port=2
  state : Inport  Port=3
  qj_des : Inport  Port=4
  CoM_Error : Inport  Port=5
  fDesQP : Inport  Port=6
  CoM_des : Inport  Port=7
  fDesNoQP : Inport  Port=8
  Enable : EnablePort
  CoM : Scope  NumInputPorts=4
  "CoM6D ->  CoMXYZ1" : Selector  NumberOfDimensions=2  InputPortWidth=7  IndexOptions=Index vector (dialog),Index vector (dialog)  Indices=[1 2 3],[1 2 3]  OutputSizes=1,1
  "CoM6D ->  CoMXYZ2" : Selector  NumberOfDimensions=2  InputPortWidth=7  IndexOptions=Index vector (dialog),Index vector (dialog)  Indices=[1 2 3],[4]  OutputSizes=1,1
  Demux : Demux  Outputs=2
  Demux3 : Demux  Outputs=2
  Demux4 : Demux  Outputs=2
  DoFs converter{,1..5} (6 alike) : WBToolboxLibrary/Utilities/DoFs converter  yarp2WBIOption=From YARP to WBI
  Gain : Gain  Gain=180/pi
  Gain3 : Gain  Gain=180/pi
  Gain4 : Gain  Gain=180/pi
  Get Measurement : WBToolboxLibrary/wholeBodyStates/Get Measurement  measuredType=Joints Torque
  Get Measurement1 : WBToolboxLibrary/wholeBodyStates/Get Measurement  measuredType=Joints Position
  Selector : Selector  NumberOfDimensions=2  IndexOptions=Index vector (dialog),Index vector (dialog)  Indices=[1:3],1  OutputSizes=1,1
  Sum : Sum  Inputs=|+-
  Sum1 : Sum  Inputs=|++
  Sum2 : Sum  Inputs=|+-
  Sum3 : Sum  Inputs=-+|
  base Pose : Scope  NumInputPorts=2
  f : Scope  NumInputPorts=7
  qj : Scope  NumInputPorts=6
  qjDes : Scope  NumInputPorts=6
  qj_err : Scope  NumInputPorts=6
  tauDes : Scope  NumInputPorts=6
  tauError : Scope  NumInputPorts=6
  tauMeasured : Scope  NumInputPorts=6
  wires:
  CoM_Error/1 -> Sum1/1, CoM/3
  CoM_des/1 -> Selector/1
  Gain/1 -> DoFs converter3/1
  Sum1/1 -> CoM/1  "CoM_Measured"
  Get Measurement1/1 -> Gain/1, Sum3/1  "qj"
  DoFs converter3/5 -> qj/5  "right_leg"
  DoFs converter3/1 -> qj/1  "torso"
  DoFs converter3/2 -> qj/2  "left_arm"
  DoFs converter3/4 -> qj/4  "left_leg"
  fDesQP/1 -> Sum2/1, Demux/1
  DoFs converter3/3 -> qj/3  "right_arm"
  Sum2/1 -> Demux3/1
  fDesNoQP/1 -> Sum2/2, Demux4/1
  tau_des/1 -> DoFs converter/1, Sum/1
  Get Measurement/1 -> DoFs converter2/1, Sum/2
  DoFs converter/5 -> tauDes/5  "right_leg"
  DoFs converter/1 -> tauDes/1  "torso"
  DoFs converter/2 -> tauDes/2  "left_arm"
  DoFs converter/4 -> tauDes/4  "left_leg"
  DoFs converter/3 -> tauDes/3  "right_arm"
  DoFs converter1/5 -> tauError/5  "right_leg"
  DoFs converter1/1 -> tauError/1  "torso"
  DoFs converter1/2 -> tauError/2  "left_arm"
  DoFs converter1/4 -> tauError/4  "left_leg"
  DoFs converter1/3 -> tauError/3  "right_arm"
  Sum/1 -> DoFs converter1/1  "torqueError"
  DoFs converter2/5 -> tauMeasured/5  "right_leg"
  DoFs converter2/1 -> tauMeasured/1  "torso"
  DoFs converter2/2 -> tauMeasured/2  "left_arm"
  DoFs converter2/4 -> tauMeasured/4  "left_leg"
  DoFs converter2/3 -> tauMeasured/3  "right_arm"
  qj_des/1 -> Sum3/2, Gain3/1
  Gain3/1 -> DoFs converter4/1
  DoFs converter4/5 -> qjDes/5  "right_leg"
  DoFs converter4/1 -> qjDes/1  "torso"
  DoFs converter4/2 -> qjDes/2  "left_arm"
  DoFs converter4/4 -> qjDes/4  "left_leg"
  DoFs converter4/3 -> qjDes/3  "right_arm"
  Gain4/1 -> DoFs converter5/1
  DoFs converter5/5 -> qj_err/5  "right_leg"
  DoFs converter5/1 -> qj_err/1  "torso"
  DoFs converter5/2 -> qj_err/2  "left_arm"
  DoFs converter5/4 -> qj_err/4  "left_leg"
  DoFs converter5/3 -> qj_err/3  "right_arm"
  Sum3/1 -> Gain4/1
  Selector/1 -> Sum1/2, CoM/2  "CoM_Desired"
  state/1 -> qj_err/6, qjDes/6, qj/6, tauDes/6, f/7, CoM/4, tauMeasured/6, tauError/6
  Demux/1 -> f/1  "wL_QP"
  Demux/2 -> f/2  "wR_QP"
  Demux3/1 -> f/3  "error_L"
  Demux3/2 -> f/4  "error_R"
  Demux4/1 -> f/5  "wL_NO_QP"
  Demux4/2 -> f/6  "wR_NO_QP"
  w_H_b/1 -> "CoM6D ->  CoMXYZ1"/1, "CoM6D ->  CoMXYZ2"/1
  "CoM6D ->  CoMXYZ2"/1 -> base Pose/1  "basePosition"
  "CoM6D ->  CoMXYZ1"/1 -> base Pose/2  "baseOrientation"

== system torqueBalancingStandup/Robot System/Dynamics and Kinematics/Dynamics ==
  w_H_b : Inport
  qj : Inport  Port=2
  nu : Inport  Port=3
  Add motors reflected inertias : Subsystem
  Centroidal Momentum : WBToolboxLibrary/wholeBodyModel/Dynamics/Centroidal Momentum
  "CoM6D ->  CoMXYZ1" : Selector  InputPortWidth=6+ROBOT_DOF  IndexOptions=Index vector (dialog)  Indices=[7:6+ROBOT_DOF]  OutputSizes=1
  "CoM6D ->  CoMXYZ2" : Selector  InputPortWidth=6+ROBOT_DOF  IndexOptions=Index vector (dialog)  Indices=[1 2 3 4 5 6]  OutputSizes=1
  Get Bias Forces : WBToolboxLibrary/wholeBodyModel/Dynamics/Get Bias Forces
  Mass Matrix : WBToolboxLibrary/wholeBodyModel/Dynamics/Mass Matrix
  M(q) : Outport
  biasTorques : Outport  Port=2
  H(q,dq) : Outport  Port=3
  wires:
  Mass Matrix/1 -> Add motors reflected inertias/1(M)
  Centroidal Momentum/1 -> H(q,dq)/1
  Get Bias Forces/1 -> biasTorques/1
  w_H_b/1 -> Centroidal Momentum/1, Get Bias Forces/1, Mass Matrix/1
  qj/1 -> Centroidal Momentum/2, Get Bias Forces/2, Mass Matrix/2
  "CoM6D ->  CoMXYZ2"/1 -> Centroidal Momentum/3, Get Bias Forces/3
  "CoM6D ->  CoMXYZ1"/1 -> Centroidal Momentum/4, Get Bias Forces/4
  nu/1 -> "CoM6D ->  CoMXYZ1"/1, "CoM6D ->  CoMXYZ2"/1
  Add motors reflected inertias/1(M_with_motor_inertia) -> M(q)/1

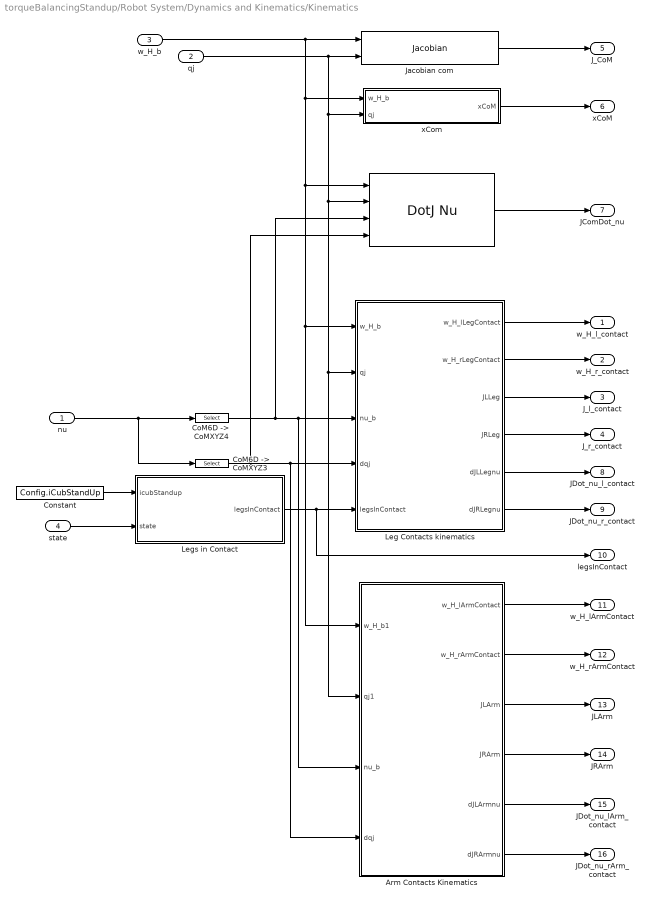
== system torqueBalancingStandup/Robot System/Dynamics and Kinematics/Kinematics ==
  nu : Inport
  qj : Inport  Port=2
  w_H_b : Inport  Port=3
  "state " : Inport  Port=4
  " " : WBToolboxLibrary/wholeBodyModel/Jacobians/DotJ Nu  frameName=Frames.COM
  Arm Contacts Kinematics : Subsystem
  "CoM6D ->  CoMXYZ3" : Selector  InputPortWidth=6+ROBOT_DOF  IndexOptions=Index vector (dialog)  Indices=[7:6+ROBOT_DOF]  OutputSizes=1
  "CoM6D ->  CoMXYZ4" : Selector  InputPortWidth=6+ROBOT_DOF  IndexOptions=Index vector (dialog)  Indices=[1 2 3 4 5 6]  OutputSizes=1
  Constant : Constant  Value=Config.iCubStandUp
  Jacobian com : WBToolboxLibrary/wholeBodyModel/Jacobians/Jacobian  frameName=Frames.COM
  Leg Contacts kinematics : Subsystem
  Legs in Contact : MATLAB Function  TreatAsAtomicUnit=on
  xCom : Subsystem
  w_H_l_contact : Outport
  w_H_r_contact : Outport  Port=2
  J_l_contact : Outport  Port=3
  J_r_contact : Outport  Port=4
  J_CoM : Outport  Port=5
  xCoM : Outport  Port=6
  JComDot_nu : Outport  Port=7
  JDot_nu_l_contact : Outport  Port=8
  JDot_nu_r_contact : Outport  Port=9
  legsInContact : Outport  Port=10
  w_H_lArmContact : Outport  Port=11
  w_H_rArmContact : Outport  Port=12
  JLArm : Outport  Port=13
  JRArm : Outport  Port=14
  JDot_nu_lArm_contact : Outport  Port=15
  JDot_nu_rArm_contact : Outport  Port=16
  wires:
  nu/1 -> "CoM6D ->  CoMXYZ3"/1, "CoM6D ->  CoMXYZ4"/1
  w_H_b/1 -> " "/1, Arm Contacts Kinematics/1(w_H_b1), Leg Contacts kinematics/1(w_H_b), xCom/1(w_H_b), Jacobian com/1
  qj/1 -> " "/2, Arm Contacts Kinematics/2(qj1), Leg Contacts kinematics/2(qj), xCom/2(qj), Jacobian com/2
  Jacobian com/1 -> J_CoM/1
  xCom/1(xCoM) -> xCoM/1
  "state "/1 -> Legs in Contact/2(state)
  Constant/1 -> Legs in Contact/1(icubStandup)
  "CoM6D ->  CoMXYZ3"/1 -> " "/4, Arm Contacts Kinematics/4(dqj), Leg Contacts kinematics/4(dqj)
  "CoM6D ->  CoMXYZ4"/1 -> " "/3, Arm Contacts Kinematics/3(nu_b), Leg Contacts kinematics/3(nu_b)
  Legs in Contact/1(legsInContact) -> Leg Contacts kinematics/5(legsInContact), legsInContact/1
  Leg Contacts kinematics/1(w_H_lLegContact) -> w_H_l_contact/1
  Leg Contacts kinematics/2(w_H_rLegContact) -> w_H_r_contact/1
  Leg Contacts kinematics/5(dJLLegnu) -> JDot_nu_l_contact/1
  Leg Contacts kinematics/6(dJRLegnu) -> JDot_nu_r_contact/1
  Leg Contacts kinematics/3(JLLeg) -> J_l_contact/1
  Leg Contacts kinematics/4(JRLeg) -> J_r_contact/1
  Arm Contacts Kinematics/1(w_H_lArmContact) -> w_H_lArmContact/1
  Arm Contacts Kinematics/2(w_H_rArmContact) -> w_H_rArmContact/1
  Arm Contacts Kinematics/3(JLArm) -> JLArm/1
  Arm Contacts Kinematics/4(JRArm) -> JRArm/1
  Arm Contacts Kinematics/5(dJLArmnu) -> JDot_nu_lArm_contact/1
  Arm Contacts Kinematics/6(dJRArmnu) -> JDot_nu_rArm_contact/1
  " "/1 -> JComDot_nu/1

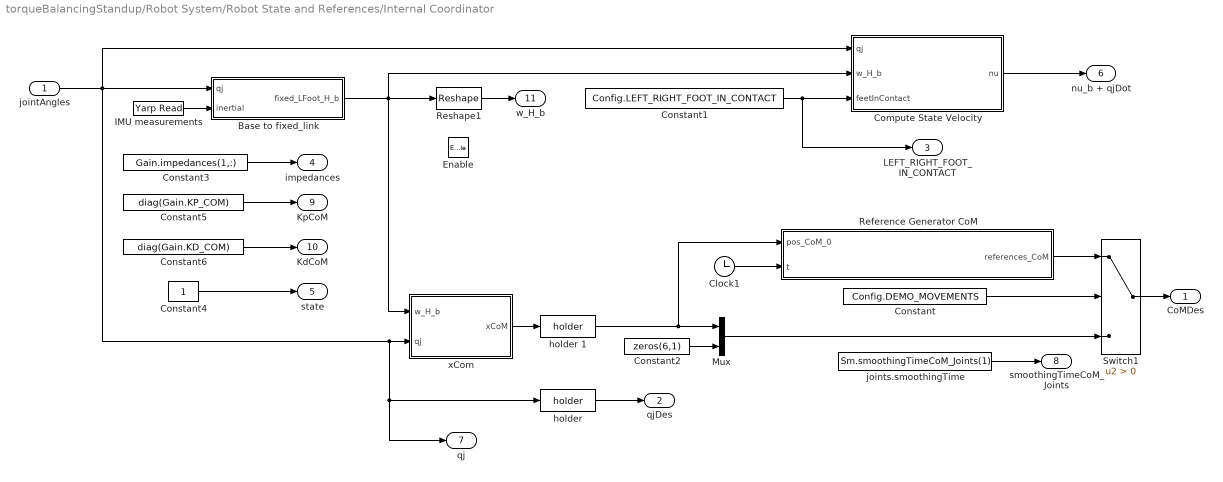
== system torqueBalancingStandup/Robot System/Robot State and References/Internal Coordinator ==
  jointAngles : Inport
  Enable : EnablePort
  Base to fixed_link : Subsystem
  Clock1 : Clock
  Compute State Velocity : Subsystem
  Constant : Constant  Value=Config.DEMO_MOVEMENTS
  Constant1 : Constant  Value=Config.LEFT_RIGHT_FOOT_IN_CONTACT
  Constant2 : Constant  Value=zeros(6,1)
  Constant3 : Constant  Value=Gain.impedances(1,:)
  Constant4 : Constant
  Constant5 : Constant  Value=diag(Gain.KP_COM)
  Constant6 : Constant  Value=diag(Gain.KD_COM)
  IMU measurements : WBToolboxLibrary/Utilities/Yarp Read  portName=Ports.IMU  signalSize=12  timeout=0.5  blocking=off  timestamp=off  autoconnect=on  errorOnConnection=on
  Mux : Mux  Inputs=2
  Reference Generator CoM : MATLAB Function  TreatAsAtomicUnit=on
  Reshape1 : Reshape  OutputDimensions=[4;4]
  Switch1 : Switch  Criteria=u2 > Threshold
  "holder " : WBToolboxLibrary/Utilities/holder 
  holder 1 : WBToolboxLibrary/Utilities/holder 
  joints.smoothingTime : Constant  Value=Sm.smoothingTimeCoM_Joints(1)
  xCom : Subsystem
  CoMDes : Outport
  qjDes : Outport  Port=2
  LEFT_RIGHT_FOOT_IN_CONTACT : Outport  Port=3
  impedances : Outport  Port=4
  state : Outport  Port=5
  nu_b + qjDot : Outport  Port=6
  qj : Outport  Port=7
  smoothingTimeCoM_Joints : Outport  Port=8
  KpCoM : Outport  Port=9
  KdCoM : Outport  Port=10
  w_H_b : Outport  Port=11
  wires:
  Constant/1 -> Switch1/2
  "holder "/1 -> qjDes/1
  Switch1/1 -> CoMDes/1
  Mux/1 -> Switch1/3
  Constant2/1 -> Mux/2
  Constant3/1 -> impedances/1
  Constant4/1 -> state/1
  Compute State Velocity/1(nu) -> nu_b + qjDot/1
  holder 1/1 -> Reference Generator CoM/1(pos_CoM_0), Mux/1
  Base to fixed_link/1(fixed_LFoot_H_b) -> Compute State Velocity/2(w_H_b), xCom/1(w_H_b), Reshape1/1
  xCom/1(xCoM) -> holder 1/1
  joints.smoothingTime/1 -> smoothingTimeCoM_Joints/1
  jointAngles/1 -> Compute State Velocity/1(qj), Base to fixed_link/1(qj), qj/1, "holder "/1, xCom/2(qj)
  Constant5/1 -> KpCoM/1
  Constant6/1 -> KdCoM/1
  Reshape1/1 -> w_H_b/1
  Constant1/1 -> Compute State Velocity/3("feetInContact "), LEFT_RIGHT_FOOT_IN_CONTACT/1
  IMU measurements/1 -> Base to fixed_link/2(inertial)
  Clock1/1 -> Reference Generator CoM/2(t)
  Reference Generator CoM/1(references_CoM) -> Switch1/1

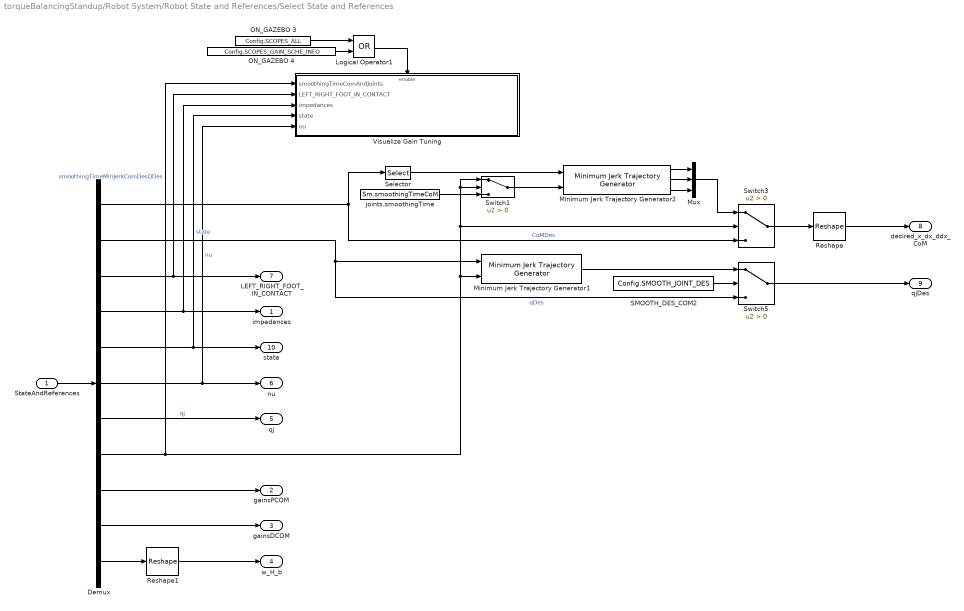
== system torqueBalancingStandup/Robot System/Robot State and References/Select State and References ==
  StateAndReferences : Inport
  Demux : Demux  Outputs=[9,ROBOT_DOF,2,ROBOT_DOF,1,ROBOT_DOF+6,ROBOT_DOF,1,3,3,16]
  Logical Operator1 : Logic  Operator=OR  AllPortsSameDT=off  OutDataTypeStr=boolean
  Minimum Jerk Trajectory Generator1 : WBToolboxLibrary/Utilities/Minimum Jerk Trajectory Generator  externalSettlingTime=on  settlingTime=1  sampleTime=Config.Ts  resetOnSettlingTime=off  firstDerivatives=off  secondDerivatives=off  explicitInitialValue=off
  Minimum Jerk Trajectory Generator2 : WBToolboxLibrary/Utilities/Minimum Jerk Trajectory Generator  externalSettlingTime=on  settlingTime=references.com.smoothingTime  sampleTime=Config.Ts  resetOnSettlingTime=off  firstDerivatives=on  secondDerivatives=on  explicitInitialValue=off
  Mux : Mux  Inputs=3
  ON_GAZEBO 3 : Constant  Value=Config.SCOPES_ALL
  ON_GAZEBO 4 : Constant  Value=Config.SCOPES_GAIN_SCHE_INFO
  Reshape : Reshape  OutputDimensionality=Customize  OutputDimensions=[3,3]
  Reshape1 : Reshape  OutputDimensionality=Customize  OutputDimensions=[4;4]
  SMOOTH_DES_COM2 : Constant  Value=Config.SMOOTH_JOINT_DES
  Selector : Selector  InputPortWidth=9  IndexOptions=Index vector (dialog)  Indices=[1 2 3]  OutputSizes=1
  Switch1 : Switch  Criteria=u2 > Threshold
  Switch3 : Switch  Criteria=u2 > Threshold
  Switch5 : Switch  Criteria=u2 > Threshold
  "Visualize Gain Tuning  " : Subsystem
  joints.smoothingTime : Constant  Value=Sm.smoothingTimeCoM
  impedances : Outport
  gainsPCOM : Outport  Port=2
  gainsDCOM : Outport  Port=3
  w_H_b : Outport  Port=4
  qj : Outport  Port=5
  nu : Outport  Port=6
  LEFT_RIGHT_FOOT_IN_CONTACT : Outport  Port=7
  desired_x_dx_ddx_CoM : Outport  Port=8
  qjDes : Outport  Port=9
  state : Outport  Port=10
  wires:
  Reshape/1 -> desired_x_dx_ddx_CoM/1
  Minimum Jerk Trajectory Generator2/1 -> Mux/1
  Minimum Jerk Trajectory Generator2/2 -> Mux/2
  Switch3/1 -> Reshape/1
  Minimum Jerk Trajectory Generator2/3 -> Mux/3
  SMOOTH_DES_COM2/1 -> Switch5/2
  Switch5/1 -> qjDes/1
  Demux/7 -> qj/1  "qj"
  Demux/11 -> Reshape1/1
  Demux/5 -> "Visualize Gain Tuning  "/4(state), state/1  "state"
  Demux/8 -> Switch1/1, Switch1/2, Switch3/2, Minimum Jerk Trajectory Generator1/2, "Visualize Gain Tuning  "/1(smoothingTimeComAndJoints)  "smoothingTimeMinJerkComDesQDes"
  Mux/1 -> Switch3/1
  Selector/1 -> Minimum Jerk Trajectory Generator2/1
  Demux/2 -> Switch5/3, Minimum Jerk Trajectory Generator1/1  "qDes"
  Minimum Jerk Trajectory Generator1/1 -> Switch5/1
  Demux/6 -> "Visualize Gain Tuning  "/5(nu), nu/1  "nu"
  StateAndReferences/1 -> Demux/1
  Demux/4 -> "Visualize Gain Tuning  "/3(impedances), impedances/1
  Demux/3 -> "Visualize Gain Tuning  "/2(LEFT_RIGHT_FOOT_IN_CONTACT), LEFT_RIGHT_FOOT_IN_CONTACT/1
  Demux/9 -> gainsPCOM/1
  Demux/10 -> gainsDCOM/1
  Demux/1 -> Selector/1, Switch3/3  "CoMDes"
  Reshape1/1 -> w_H_b/1
  ON_GAZEBO 4/1 -> Logical Operator1/2
  ON_GAZEBO 3/1 -> Logical Operator1/1
  Logical Operator1/1 -> "Visualize Gain Tuning  "/Enable
  Switch1/1 -> Minimum Jerk Trajectory Generator2/2
  joints.smoothingTime/1 -> Switch1/3
